simulink model "unver4"  (R2020b)
settings: Solver=ode45  StartTime=0.0  StopTime=50  FixedStep=0.001  RelTol=1e-3
undefined symbols (not defined in the file): c1, c2, c3, c4, fn, jw, m, r
settings Model: Creator=K E S SRINIVAS  LastModifiedBy=K E S SRINIVAS
settings SolverCC: ZeroCrossAlgorithm=Adaptive

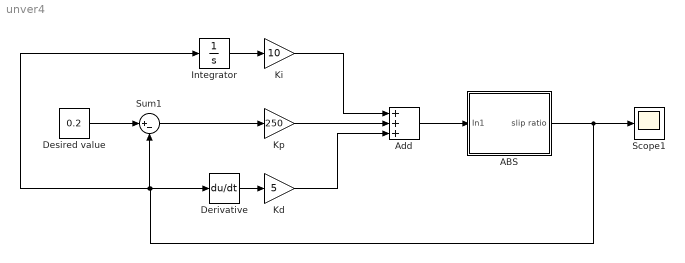
== system unver4 ==
  ABS : Subsystem
  Add : Sum  Inputs=+++
  Derivative : Derivative
  Desired value : Constant  Value=0.2
  Integrator : Integrator
  Kd : Gain  Gain=5
  Ki : Gain  Gain=10
  Kp : Gain  Gain=250
  Scope1 : Scope
  Sum1 : Sum  Inputs=|+-
  wires:
  ABS/1(slip ratio) -> Sum1/2, Integrator/1, Derivative/1, Scope1/1
  Add/1 -> ABS/1(In1)
  Ki/1 -> Add/1
  Integrator/1 -> Ki/1
  Kp/1 -> Add/2
  Sum1/1 -> Kp/1
  Desired value/1 -> Sum1/1
  Derivative/1 -> Kd/1
  Kd/1 -> Add/3

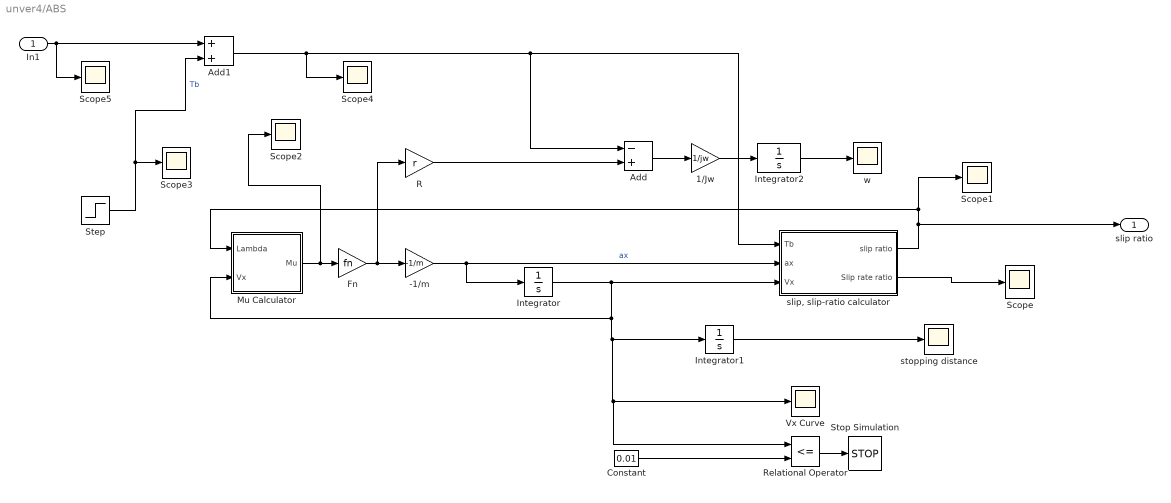
== system unver4/ABS ==
  In1 : Inport
  -1/m : Gain  Gain=-1/m
  1/Jw : Gain  Gain=1/jw
  Add : Sum  Inputs=-+
  Add1 : Sum
  Constant : Constant  Value=0.01
  Fn : Gain  Gain=fn
  Integrator : Integrator  InitialCondition=27.78  LimitOutput=on  UpperSaturationLimit=27.78  LowerSaturationLimit=0
  Integrator1 : Integrator  LowerSaturationLimit=0
  Integrator2 : Integrator  InitialCondition=84.18  LimitOutput=on  LowerSaturationLimit=0
  Mu Calculator : Subsystem
  R : Gain  Gain=r
  Relational Operator : RelationalOperator  Operator=<=  OutDataTypeStr=boolean  RndMeth=Simplest
  Scope{,1..5} (6 alike) : Scope
  Step : Step  Time=0  After=1200  SampleTime=0
  Stop Simulation : Stop
  Vx Curve : Scope
  "slip, slip-ratio calculator" : Subsystem
  stopping distance : Scope
  w : Scope
  slip ratio : Outport
  wires:
  Mu Calculator/1(Mu) -> Scope2/1, Fn/1
  Integrator/1 -> Relational Operator/1, Vx Curve/1, Integrator1/1, Mu Calculator/2(Vx), "slip, slip-ratio calculator"/3(Vx)
  -1/m/1 -> Integrator/1, "slip, slip-ratio calculator"/2(ax)  "ax"
  "slip, slip-ratio calculator"/1(slip ratio) -> Scope1/1, Mu Calculator/1(Lambda), slip ratio/1
  Relational Operator/1 -> Stop Simulation/1
  Constant/1 -> Relational Operator/2
  Integrator1/1 -> stopping distance/1
  Add1/1 -> Scope4/1, Add/1, "slip, slip-ratio calculator"/1(Tb)
  Fn/1 -> R/1, -1/m/1
  R/1 -> Add/2
  Add/1 -> 1/Jw/1
  "slip, slip-ratio calculator"/2(Slip rate ratio) -> Scope/1
  1/Jw/1 -> Integrator2/1
  Integrator2/1 -> w/1
  In1/1 -> Scope5/1, Add1/1
  Step/1 -> Add1/2, Scope3/1  "Tb"

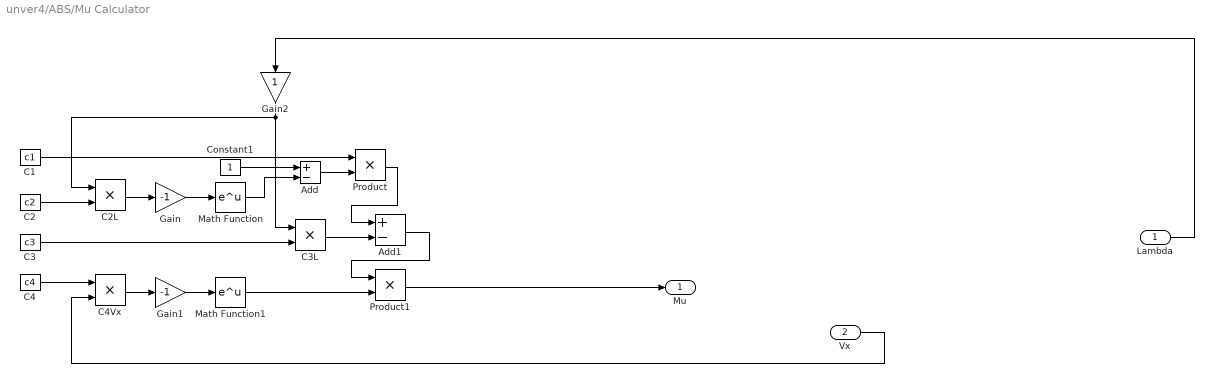
== system unver4/ABS/Mu Calculator ==
  Lambda : Inport
  Vx : Inport  Port=2
  Add : Sum  Inputs=+-
  Add1 : Sum  Inputs=+-
  C1 : Constant  Value=c1
  C2 : Constant  Value=c2
  C2L : Product
  C3 : Constant  Value=c3
  C3L : Product
  C4 : Constant  Value=c4
  C4Vx : Product
  Constant1 : Constant
  Gain : Gain  Gain=-1
  Gain1 : Gain  Gain=-1
  Gain2 : Gain
  Math Function : Math  SaturateOnIntegerOverflow=on
  Math Function1 : Math  SaturateOnIntegerOverflow=on
  Product : Product
  Product1 : Product
  Mu : Outport
  wires:
  C2/1 -> C2L/2
  Gain/1 -> Math Function/1
  C1/1 -> Product/1
  C2L/1 -> Gain/1
  Constant1/1 -> Add/1
  Vx/1 -> C4Vx/2
  C4/1 -> C4Vx/1
  Add/1 -> Product/2
  Math Function/1 -> Add/2
  Gain1/1 -> Math Function1/1
  Math Function1/1 -> Product1/2
  C3L/1 -> Add1/2
  Gain2/1 -> C3L/1, C2L/1
  Product1/1 -> Mu/1
  C4Vx/1 -> Gain1/1
  C3/1 -> C3L/2
  Product/1 -> Add1/1
  Add1/1 -> Product1/1
  Lambda/1 -> Gain2/1

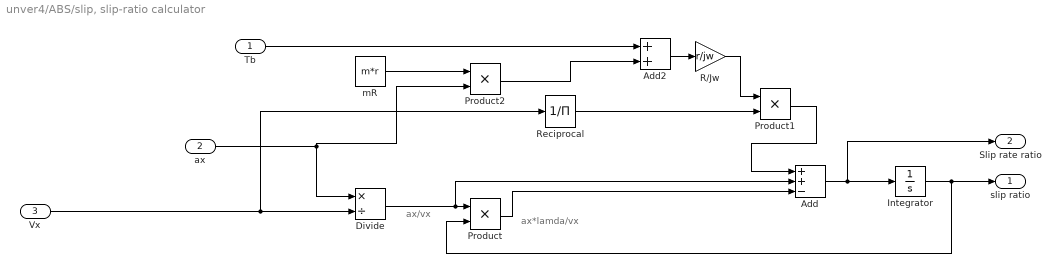
== system unver4/ABS/slip, slip-ratio calculator ==
  note: ax*lamda/vx
  note: ax/vx
  Tb : Inport
  ax : Inport  Port=2
  Vx : Inport  Port=3
  Add : Sum  Inputs=++-
  Add2 : Sum
  Divide : Product  Inputs=*/
  Integrator : Integrator  UpperSaturationLimit=1  LowerSaturationLimit=0
  Product : Product
  Product1 : Product
  Product2 : Product
  R/Jw : Gain  Gain=r/jw
  Reciprocal : Product  Inputs=/
  mR : Constant  Value=m*r
  slip ratio : Outport
  Slip rate ratio : Outport  Port=2
  wires:
  ax/1 -> Divide/1, Product2/2
  Divide/1 -> Add/2, Product/1
  Product1/1 -> Add/1
  Product/1 -> Add/3
  Add/1 -> Slip rate ratio/1, Integrator/1
  R/Jw/1 -> Product1/1
  Tb/1 -> Add2/1
  Integrator/1 -> Product/2, slip ratio/1
  mR/1 -> Product2/1
  Product2/1 -> Add2/2
  Add2/1 -> R/Jw/1
  Vx/1 -> Reciprocal/1, Divide/2
  Reciprocal/1 -> Product1/2
